simulink model "FINAL_DC_MULTIGUN_CHARGER_NEW"  (R2021b)
settings: Solver=FixedStepDiscrete  StartTime=0.0  StopTime=3600  FixedStep=0.1  RelTol=1e-3
model workspace (MAT data in the model file):
  P.stn.Ptotal_kW = 180
  P.stn.Nmod = 6
  P.stn.Pmod_kW = 30
  P.stn.Nev = 3
  P.stn.PgunMax_kW = 120
  P.stn.NmodGunMax = 4
  P.stn.Vbus_nom = 800
  P.ts.fast = 0.1
  P.ts.sup = 1
  P.tstop = 3600
  P.socStop = 0.97
  P.socMin = 0.1
  P.ev.Cap_kWh = [60 80 50]
  P.ev.Vnom = [500 560 480]
  P.ev.Vmax = [650 700 640]
  P.ev.Imax_A = [200 150 180]
  P.ev.Pmax_kW = [80 120 60]
  P.ev.Rint = [0.06 0.08 0.07]
  P.ev.SOC0 = [0.15 0.3 0.55]
  P.ev.Temp0 = [30 38 35]
  P.bms1 = '[60;500;650;200;80;0.06;30]'
  P.bms2 = '[80;560;700;150;120;0.08;38]'
  P.bms3 = '[50;480;640;180;60;0.07;35]'
  P.soc0 = [0.15; 0.3; 0.55]
  P.w.SOC = 0.35
  P.w.Demand = 0.25
  P.w.Urg = 0.25
  P.w.Fair = 0.15
  P.th.Cth = 60000
  P.th.Rth = 0.01
  P.th.Tamb = 25
  P.th.WARM = 40
  P.th.HOT = 50
  P.th.PROT = 55
  P.sw.tRampDown = 1
  P.sw.tOpenDelay = 0.2
  P.sw.tDeadTime = 0.5
  P.sw.tConnect = 0.2
  P.sw.tRampUp = 1
  P.mode = 5
  P.scenario = 2
  P.faultSchedule = 'zeros(0,4)'
settings Model: Creator=ratan  LastModifiedBy=ratan

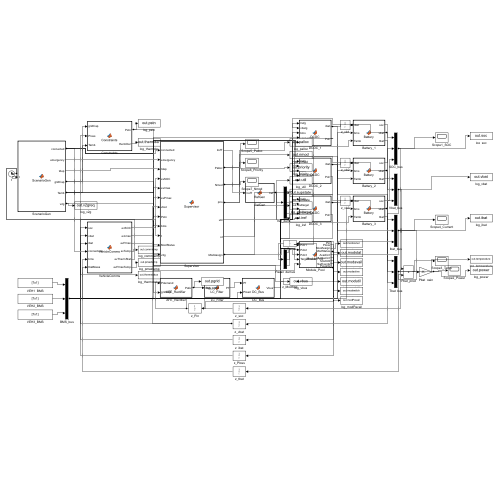
[thumbnail: Simulink's stored preview of the top-level diagram]
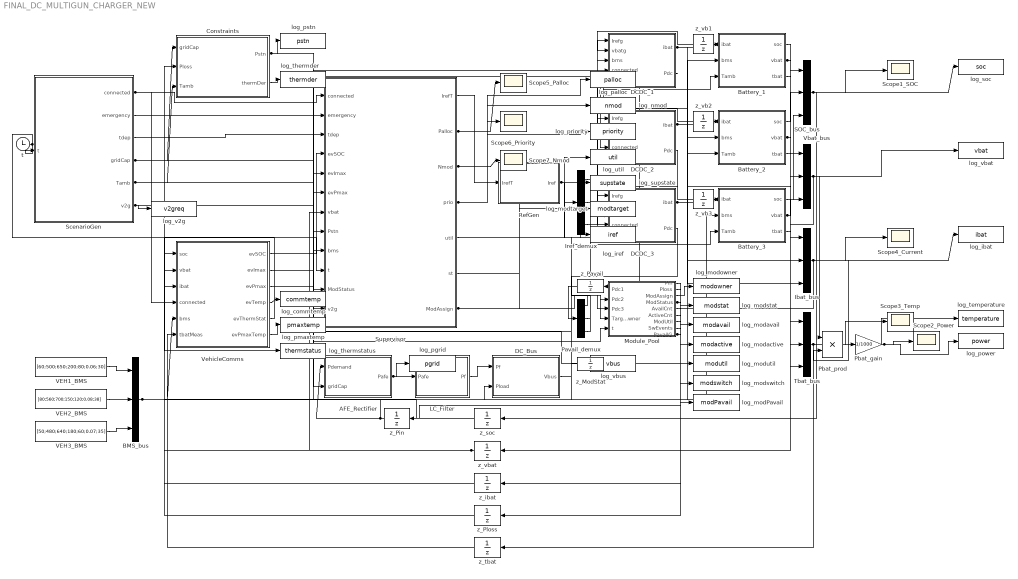
== system FINAL_DC_MULTIGUN_CHARGER_NEW ==
  AFE_Rectifier : MATLAB Function  TreatAsAtomicUnit=on
  BMS_bus : Mux  Inputs=3
  Battery_1 : MATLAB Function  TreatAsAtomicUnit=on
  Battery_2 : MATLAB Function  TreatAsAtomicUnit=on
  Battery_3 : MATLAB Function  TreatAsAtomicUnit=on
  Constraints : MATLAB Function  TreatAsAtomicUnit=on
  DCDC_1 : MATLAB Function  TreatAsAtomicUnit=on
  DCDC_2 : MATLAB Function  TreatAsAtomicUnit=on
  DCDC_3 : MATLAB Function  TreatAsAtomicUnit=on
  DC_Bus : MATLAB Function  TreatAsAtomicUnit=on
  Ibat_bus : Mux  Inputs=3
  Iref_demux : Demux  Outputs=3
  LC_Filter : MATLAB Function  TreatAsAtomicUnit=on
  Module_Pool : MATLAB Function  TreatAsAtomicUnit=on
  Pavail_demux : Demux  Outputs=3
  Pbat_gain : Gain  Gain=1/1000
  Pbat_prod : Product
  RefGen : MATLAB Function  TreatAsAtomicUnit=on
  SOC_bus : Mux  Inputs=3
  ScenarioGen : MATLAB Function  TreatAsAtomicUnit=on
  Scope1_SOC : Scope
  Scope2_Power : Scope
  Scope3_Temp : Scope
  Scope4_Current : Scope
  Scope5_Palloc : Scope
  Scope6_Priority : Scope
  Scope7_Nmod : Scope
  Supervisor : MATLAB Function  TreatAsAtomicUnit=on
  Tbat_bus : Mux  Inputs=3
  VEH1_BMS : Constant  Value=[60;500;650;200;80;0.06;30]
  VEH2_BMS : Constant  Value=[80;560;700;150;120;0.08;38]
  VEH3_BMS : Constant  Value=[50;480;640;180;60;0.07;35]
  Vbat_bus : Mux  Inputs=3
  VehicleComms : MATLAB Function  TreatAsAtomicUnit=on
  log_commtemp : ToWorkspace  VariableName=commtemp  SaveFormat=Timeseries  SampleTime=-1
  log_ibat : ToWorkspace  VariableName=ibat  SaveFormat=Timeseries  SampleTime=-1
  log_iref : ToWorkspace  VariableName=iref  SaveFormat=Timeseries  SampleTime=-1
  log_modPavail : ToWorkspace  VariableName=modPavail  SaveFormat=Timeseries  SampleTime=-1
  log_modactive : ToWorkspace  VariableName=modactive  SaveFormat=Timeseries  SampleTime=-1
  log_modavail : ToWorkspace  VariableName=modavail  SaveFormat=Timeseries  SampleTime=-1
  log_modowner : ToWorkspace  VariableName=modowner  SaveFormat=Timeseries  SampleTime=-1
  log_modstat : ToWorkspace  VariableName=modstat  SaveFormat=Timeseries  SampleTime=-1
  log_modswitch : ToWorkspace  VariableName=modswitch  SaveFormat=Timeseries  SampleTime=-1
  log_modtarget : ToWorkspace  VariableName=modtarget  SaveFormat=Timeseries  SampleTime=-1
  log_modutil : ToWorkspace  VariableName=modutil  SaveFormat=Timeseries  SampleTime=-1
  log_nmod : ToWorkspace  VariableName=nmod  SaveFormat=Timeseries  SampleTime=-1
  log_palloc : ToWorkspace  VariableName=palloc  SaveFormat=Timeseries  SampleTime=-1
  log_pgrid : ToWorkspace  VariableName=pgrid  SaveFormat=Timeseries  SampleTime=-1
  log_pmaxtemp : ToWorkspace  VariableName=pmaxtemp  SaveFormat=Timeseries  SampleTime=-1
  log_power : ToWorkspace  VariableName=power  SaveFormat=Timeseries  SampleTime=-1
  log_priority : ToWorkspace  VariableName=priority  SaveFormat=Timeseries  SampleTime=-1
  log_pstn : ToWorkspace  VariableName=pstn  SaveFormat=Timeseries  SampleTime=-1
  log_soc : ToWorkspace  VariableName=soc  SaveFormat=Timeseries  SampleTime=-1
  log_supstate : ToWorkspace  VariableName=supstate  SaveFormat=Timeseries  SampleTime=-1
  log_temperature : ToWorkspace  VariableName=temperature  SaveFormat=Timeseries  SampleTime=-1
  log_thermder : ToWorkspace  VariableName=thermder  SaveFormat=Timeseries  SampleTime=-1
  log_thermstatus : ToWorkspace  VariableName=thermstatus  SaveFormat=Timeseries  SampleTime=-1
  log_util : ToWorkspace  VariableName=util  SaveFormat=Timeseries  SampleTime=-1
  log_v2g : ToWorkspace  VariableName=v2greq  SaveFormat=Timeseries  SampleTime=-1
  log_vbat : ToWorkspace  VariableName=vbat  SaveFormat=Timeseries  SampleTime=-1
  log_vbus : ToWorkspace  VariableName=vbus  SaveFormat=Timeseries  SampleTime=-1
  t : Clock
  z_ModStat : UnitDelay  InitialCondition=[0;0;0;0;0;0]  SampleTime=0.1  HasFrameUpgradeWarning=on
  z_Pavail : UnitDelay  InitialCondition=[0;0;0]  SampleTime=0.1  HasFrameUpgradeWarning=on
  z_Pin : UnitDelay  SampleTime=0.1  HasFrameUpgradeWarning=on
  z_Ploss : UnitDelay  SampleTime=0.1  HasFrameUpgradeWarning=on
  z_ibat : UnitDelay  InitialCondition=[0;0;0]  SampleTime=0.1  HasFrameUpgradeWarning=on
  z_soc : UnitDelay  InitialCondition=[0.15;0.3;0.55]  SampleTime=0.1  HasFrameUpgradeWarning=on
  z_tbat : UnitDelay  InitialCondition=[30;38;35]  SampleTime=0.1  HasFrameUpgradeWarning=on
  z_vb1 : UnitDelay  InitialCondition=500  SampleTime=0.1  HasFrameUpgradeWarning=on
  z_vb2 : UnitDelay  InitialCondition=560  SampleTime=0.1  HasFrameUpgradeWarning=on
  z_vb3 : UnitDelay  InitialCondition=480  SampleTime=0.1  HasFrameUpgradeWarning=on
  z_vbat : UnitDelay  InitialCondition=[500;560;480]  SampleTime=0.1  HasFrameUpgradeWarning=on
  wires:
  VEH1_BMS/1 -> BMS_bus/1
  VEH2_BMS/1 -> BMS_bus/2
  VEH3_BMS/1 -> BMS_bus/3
  t/1 -> ScenarioGen/1(t), Supervisor/10(t), Module_Pool/5(t)
  ScenarioGen/1(connected) -> Supervisor/1(connected), VehicleComms/4(connected), DCDC_1/4(connected), DCDC_2/4(connected), DCDC_3/4(connected)
  ScenarioGen/2(emergency) -> Supervisor/2(emergency)
  ScenarioGen/3(tdep) -> Supervisor/3(tdep)
  ScenarioGen/6(v2g) -> Supervisor/12(v2g), log_v2g/1
  ScenarioGen/4(gridCap) -> Constraints/1(gridCap), AFE_Rectifier/2(gridCap)
  ScenarioGen/5(Tamb) -> Constraints/3(Tamb), Battery_1/3(Tamb), Battery_2/3(Tamb), Battery_3/3(Tamb)
  z_soc/1 -> VehicleComms/1(soc)
  z_vbat/1 -> VehicleComms/2(vbat), Supervisor/7(vbat)
  z_ibat/1 -> VehicleComms/3(ibat)
  BMS_bus/1 -> VehicleComms/5(bms), Supervisor/9(bms), DCDC_1/3(bms), Battery_1/2(bms), DCDC_2/3(bms), Battery_2/2(bms), DCDC_3/3(bms), Battery_3/2(bms)
  z_tbat/1 -> VehicleComms/6(tbatMeas)
  z_Ploss/1 -> Constraints/2(Ploss)
  VehicleComms/1(evSOC) -> Supervisor/4(evSOC)
  VehicleComms/2(evImax) -> Supervisor/5(evImax)
  VehicleComms/3(evPmax) -> Supervisor/6(evPmax)
  Constraints/1(Pstn) -> Supervisor/8(Pstn), log_pstn/1
  z_ModStat/1 -> Supervisor/11(ModStatus)
  Supervisor/1(IrefT) -> RefGen/1(IrefT)
  RefGen/1(Iref) -> Iref_demux/1, log_iref/1
  Iref_demux/1 -> DCDC_1/1(Irefg)
  Iref_demux/2 -> DCDC_2/1(Irefg)
  Iref_demux/3 -> DCDC_3/1(Irefg)
  Supervisor/7(ModAssign) -> Module_Pool/4(TargetOwner), log_modtarget/1
  Battery_1/2(vbat) -> z_vb1/1, Vbat_bus/1
  z_vb1/1 -> DCDC_1/2(vbatg)
  Battery_2/2(vbat) -> z_vb2/1, Vbat_bus/2
  z_vb2/1 -> DCDC_2/2(vbatg)
  Battery_3/2(vbat) -> z_vb3/1, Vbat_bus/3
  z_vb3/1 -> DCDC_3/2(vbatg)
  Pavail_demux/1 -> DCDC_1/5(Pavail)
  Pavail_demux/2 -> DCDC_2/5(Pavail)
  Pavail_demux/3 -> DCDC_3/5(Pavail)
  DCDC_1/1(ibat) -> Battery_1/1(ibat), Ibat_bus/1
  DCDC_2/1(ibat) -> Battery_2/1(ibat), Ibat_bus/2
  DCDC_3/1(ibat) -> Battery_3/1(ibat), Ibat_bus/3
  Battery_1/1(soc) -> SOC_bus/1
  Battery_2/1(soc) -> SOC_bus/2
  Battery_3/1(soc) -> SOC_bus/3
  SOC_bus/1 -> z_soc/1, Scope1_SOC/1, log_soc/1
  Vbat_bus/1 -> z_vbat/1, Pbat_prod/1, log_vbat/1
  Ibat_bus/1 -> z_ibat/1, Pbat_prod/2, Scope4_Current/1, log_ibat/1
  Battery_1/3(tbat) -> Tbat_bus/1
  Battery_2/3(tbat) -> Tbat_bus/2
  Battery_3/3(tbat) -> Tbat_bus/3
  Tbat_bus/1 -> z_tbat/1, Scope3_Temp/1, log_temperature/1
  Pbat_prod/1 -> Pbat_gain/1
  DCDC_1/2(Pdc) -> Module_Pool/1(Pdc1)
  DCDC_2/2(Pdc) -> Module_Pool/2(Pdc2)
  DCDC_3/2(Pdc) -> Module_Pool/3(Pdc3)
  Module_Pool/1(Pin) -> z_Pin/1
  Module_Pool/2(Ploss) -> z_Ploss/1
  Module_Pool/4(ModStatus) -> z_ModStat/1, log_modstat/1
  Module_Pool/9(PavailG) -> z_Pavail/1, log_modPavail/1
  z_Pavail/1 -> Pavail_demux/1
  z_Pin/1 -> AFE_Rectifier/1(Pdemand), DC_Bus/2(Pload)
  AFE_Rectifier/1(Pafe) -> LC_Filter/1(Pafe), log_pgrid/1
  LC_Filter/1(Pf) -> DC_Bus/1(Pf)
  Pbat_gain/1 -> Scope2_Power/1, log_power/1
  Supervisor/2(Palloc) -> Scope5_Palloc/1, log_palloc/1
  Supervisor/4(prio) -> Scope6_Priority/1, log_priority/1
  Supervisor/3(Nmod) -> Scope7_Nmod/1, log_nmod/1
  Supervisor/5(util) -> log_util/1
  Supervisor/6(st) -> log_supstate/1
  VehicleComms/6(evPmaxTemp) -> log_pmaxtemp/1
  VehicleComms/5(evThermStat) -> log_thermstatus/1
  VehicleComms/4(evTemp) -> log_commtemp/1
  Constraints/2(thermDer) -> log_thermder/1
  DC_Bus/1(Vbus) -> log_vbus/1
  Module_Pool/3(ModAssign) -> log_modowner/1
  Module_Pool/5(AvailCnt) -> log_modavail/1
  Module_Pool/6(ActiveCnt) -> log_modactive/1
  Module_Pool/7(ModUtil) -> log_modutil/1
  Module_Pool/8(SwEvents) -> log_modswitch/1

== matlab function FINAL_DC_MULTIGUN_CHARGER_NEW/DCDC_2 ==
  data: Irefg input; ibat output; vbatg input; bms input; connected input; Pavail input; Pdc output
function [ibat,Pdc] = DCDC(Irefg,vbatg,bms,connected,Pavail)
%#codegen
G_INJECT=2; g=G_INJECT; o=(g-1)*7;
Vmax=bms(o+3); Rint=bms(o+6); Imax=bms(o+4);
Ts=0.1; tauI=0.08; persistent I; if isempty(I), I=0; end
Icap=Pavail*1000/max(vbatg,100);
if Irefg >= 0
  Icv=max(I+(Vmax-vbatg)/max(Rint,1e-3),0);
  Icmd=min([Irefg,Icv,Icap]);
else
  Icmd=max([Irefg,-Icap,-Imax]);   % V2G discharge, magnitude-limited
end
Icmd=Icmd*(connected(g)>0.5);
I=I+(Ts/tauI)*(Icmd-I);
ibat=I; Pdc=vbatg*I/1000;
end

== matlab function FINAL_DC_MULTIGUN_CHARGER_NEW/DCDC_3 ==
  data: Irefg input; ibat output; vbatg input; bms input; connected input; Pavail input; Pdc output
function [ibat,Pdc] = DCDC(Irefg,vbatg,bms,connected,Pavail)
%#codegen
G_INJECT=3; g=G_INJECT; o=(g-1)*7;
Vmax=bms(o+3); Rint=bms(o+6); Imax=bms(o+4);
Ts=0.1; tauI=0.08; persistent I; if isempty(I), I=0; end
Icap=Pavail*1000/max(vbatg,100);
if Irefg >= 0
  Icv=max(I+(Vmax-vbatg)/max(Rint,1e-3),0);
  Icmd=min([Irefg,Icv,Icap]);
else
  Icmd=max([Irefg,-Icap,-Imax]);   % V2G discharge, magnitude-limited
end
Icmd=Icmd*(connected(g)>0.5);
I=I+(Ts/tauI)*(Icmd-I);
ibat=I; Pdc=vbatg*I/1000;
end

== matlab function FINAL_DC_MULTIGUN_CHARGER_NEW/Battery_1 ==
  data: ibat input; soc output; bms input; Tamb input; vbat output; tbat output
function [soc,vbat,tbat] = Battery(ibat,bms,Tamb)
%#codegen
G_INJECT=1; g=G_INJECT; o=(g-1)*7;
SOC0_INJECT=0.15; TBAT0_INJECT=30; CTH_INJECT=60000; RTH_INJECT=0.01;
Cap_kWh=bms(o+1); Vnom=bms(o+2); Vmax=bms(o+3); Rint=bms(o+6);
% initial SOC and initial pack temperature are scenario INITIAL CONDITIONS
% injected at build time (ov.soc0 / ov.temp0) - deliberately NOT taken from
% the runtime BMS panel, so editing VEH*_BMS cannot move the start state.
Ts=0.1; persistent SOC Tb; if isempty(SOC), SOC=SOC0_INJECT; Tb=TBAT0_INJECT; end
Ah=Cap_kWh*1000/max(Vnom,100);
SOC=min(max(SOC+ibat*Ts/3600/Ah,0),1);   % charge + discharge (V2G)
ocv=Vnom*(0.86+0.10*SOC+0.10*max(SOC-0.8,0)/0.2);
V=ocv+ibat*Rint; if V>Vmax, V=Vmax; end; if V<0.5*Vnom, V=0.5*Vnom; end
Ploss=ibat*ibat*Rint;
Tb=Tb+Ts*(Ploss-(Tb-Tamb)/max(RTH_INJECT,1e-6))/max(CTH_INJECT,1e-6);
if Tb<-30, Tb=-30; end; if Tb>90, Tb=90; end
soc=SOC; vbat=V; tbat=Tb;
end

== matlab function FINAL_DC_MULTIGUN_CHARGER_NEW/Battery_2 ==
  data: ibat input; soc output; bms input; Tamb input; vbat output; tbat output
function [soc,vbat,tbat] = Battery(ibat,bms,Tamb)
%#codegen
G_INJECT=2; g=G_INJECT; o=(g-1)*7;
SOC0_INJECT=0.3; TBAT0_INJECT=38; CTH_INJECT=60000; RTH_INJECT=0.01;
Cap_kWh=bms(o+1); Vnom=bms(o+2); Vmax=bms(o+3); Rint=bms(o+6);
% initial SOC and initial pack temperature are scenario INITIAL CONDITIONS
% injected at build time (ov.soc0 / ov.temp0) - deliberately NOT taken from
% the runtime BMS panel, so editing VEH*_BMS cannot move the start state.
Ts=0.1; persistent SOC Tb; if isempty(SOC), SOC=SOC0_INJECT; Tb=TBAT0_INJECT; end
Ah=Cap_kWh*1000/max(Vnom,100);
SOC=min(max(SOC+ibat*Ts/3600/Ah,0),1);   % charge + discharge (V2G)
ocv=Vnom*(0.86+0.10*SOC+0.10*max(SOC-0.8,0)/0.2);
V=ocv+ibat*Rint; if V>Vmax, V=Vmax; end; if V<0.5*Vnom, V=0.5*Vnom; end
Ploss=ibat*ibat*Rint;
Tb=Tb+Ts*(Ploss-(Tb-Tamb)/max(RTH_INJECT,1e-6))/max(CTH_INJECT,1e-6);
if Tb<-30, Tb=-30; end; if Tb>90, Tb=90; end
soc=SOC; vbat=V; tbat=Tb;
end

== matlab function FINAL_DC_MULTIGUN_CHARGER_NEW/Battery_3 ==
  data: ibat input; soc output; bms input; Tamb input; vbat output; tbat output
function [soc,vbat,tbat] = Battery(ibat,bms,Tamb)
%#codegen
G_INJECT=3; g=G_INJECT; o=(g-1)*7;
SOC0_INJECT=0.55; TBAT0_INJECT=35; CTH_INJECT=60000; RTH_INJECT=0.01;
Cap_kWh=bms(o+1); Vnom=bms(o+2); Vmax=bms(o+3); Rint=bms(o+6);
% initial SOC and initial pack temperature are scenario INITIAL CONDITIONS
% injected at build time (ov.soc0 / ov.temp0) - deliberately NOT taken from
% the runtime BMS panel, so editing VEH*_BMS cannot move the start state.
Ts=0.1; persistent SOC Tb; if isempty(SOC), SOC=SOC0_INJECT; Tb=TBAT0_INJECT; end
Ah=Cap_kWh*1000/max(Vnom,100);
SOC=min(max(SOC+ibat*Ts/3600/Ah,0),1);   % charge + discharge (V2G)
ocv=Vnom*(0.86+0.10*SOC+0.10*max(SOC-0.8,0)/0.2);
V=ocv+ibat*Rint; if V>Vmax, V=Vmax; end; if V<0.5*Vnom, V=0.5*Vnom; end
Ploss=ibat*ibat*Rint;
Tb=Tb+Ts*(Ploss-(Tb-Tamb)/max(RTH_INJECT,1e-6))/max(CTH_INJECT,1e-6);
if Tb<-30, Tb=-30; end; if Tb>90, Tb=90; end
soc=SOC; vbat=V; tbat=Tb;
end

== matlab function FINAL_DC_MULTIGUN_CHARGER_NEW/Module_Pool ==
  data: Pdc1 input; Pin output; Pdc2 input; Pdc3 input; TargetOwner input; t input; Ploss output; ModAssign output; ModStatus output; AvailCnt output; ActiveCnt output; ModUtil output; SwEvents output; PavailG output
function [Pin,Ploss,ModAssign,ModStatus,AvailCnt,ActiveCnt,ModUtil,SwEvents,PavailG] = ModulePool(Pdc1,Pdc2,Pdc3,TargetOwner,t)
%#codegen
Pmod=30; eta=0.955; SWLOSS_KW=0.3;
TRD_M=1; TOPEN_M=0.2; TDEAD_M=0.5; TCONN_M=0.2; TRUP_M=1;
FAULT_SCHEDULE=zeros(0,4); Ts=0.1;
persistent owner phase timer contrib pend swCnt initMP;
if isempty(initMP), owner=zeros(6,1); phase=zeros(6,1); timer=zeros(6,1); contrib=zeros(6,1); pend=zeros(6,1); swCnt=0; initMP=1; end
health=zeros(6,1);
for r=1:size(FAULT_SCHEDULE,1), mid=FAULT_SCHEDULE(r,1); if t>=FAULT_SCHEDULE(r,2) && t<=FAULT_SCHEDULE(r,3), health(mid)=FAULT_SCHEDULE(r,4); end, end
for id=1:6
  tgt=TargetOwner(id);
  if health(id)~=0
    owner(id)=0; pend(id)=0; contrib(id)=0;
    if phase(id)~=0, timer(id)=timer(id)+Ts; if timer(id)>=TDEAD_M, phase(id)=0; timer(id)=0; end, end
  else
    switch phase(id)
      case 0, if tgt>0, pend(id)=tgt; phase(id)=5; timer(id)=0; end
      case 1, if tgt~=owner(id), pend(id)=tgt; phase(id)=2; timer(id)=0; end
      case 2, timer(id)=timer(id)+Ts; contrib(id)=max(1-timer(id)/max(TRD_M,1e-3),0); if timer(id)>=TRD_M, phase(id)=3; timer(id)=0; contrib(id)=0; end
      case 3, timer(id)=timer(id)+Ts; if timer(id)>=TOPEN_M, owner(id)=0; phase(id)=4; timer(id)=0; end
      case 4, timer(id)=timer(id)+Ts; if timer(id)>=TDEAD_M, if pend(id)>0, phase(id)=5; timer(id)=0; else phase(id)=0; timer(id)=0; end, end
      case 5, timer(id)=timer(id)+Ts; if timer(id)>=TCONN_M, owner(id)=pend(id); pend(id)=0; phase(id)=6; timer(id)=0; end
      case 6, timer(id)=timer(id)+Ts; contrib(id)=min(timer(id)/max(TRUP_M,1e-3),1); if timer(id)>=TRUP_M, phase(id)=1; timer(id)=0; contrib(id)=1; swCnt=swCnt+1; end
    end
  end
end
ModAssign=owner; ModUtil=contrib; ModStatus=zeros(6,1);
for id=1:6, if health(id)~=0, ModStatus(id)=health(id)+1; elseif phase(id)==0, ModStatus(id)=0; else ModStatus(id)=1; end, end
AvailCnt=sum(ModStatus==0); ActiveCnt=sum(phase>0 & health==0); SwEvents=swCnt;
PavailG=zeros(3,1); for id=1:6, gg=owner(id); if gg>0, PavailG(gg)=PavailG(gg)+contrib(id)*Pmod; end, end
nTrans=sum(phase>=2 & phase<=5 & health==0);
Pdc=Pdc1+Pdc2+Pdc3;
if Pdc>=0, Pin=Pdc/eta+SWLOSS_KW*nTrans; else Pin=Pdc*eta+SWLOSS_KW*nTrans; end
Ploss=abs(Pin-Pdc);
end

== matlab function FINAL_DC_MULTIGUN_CHARGER_NEW/AFE_Rectifier ==
  data: Pdemand input; Pafe output; gridCap input
function Pafe = AFE_Rectifier(Pdemand,gridCap)
%#codegen
Ts=0.1; SLEW=60; persistent P; if isempty(P), P=0; end
tgt=min(Pdemand,gridCap);   % gridCap limits import; export (negative) passes
P=P+max(min(tgt-P,SLEW*Ts),-SLEW*Ts);
Pafe=P;   % may be negative (V2G export to grid)
end

== matlab function FINAL_DC_MULTIGUN_CHARGER_NEW/LC_Filter ==
  data: Pafe input; Pf output
function Pf = LC_Filter(Pafe)
%#codegen
Ts=0.1; tau=0.3; persistent P; if isempty(P), P=0; end
P=P+(Ts/tau)*(Pafe-P); Pf=P;
end

== matlab function FINAL_DC_MULTIGUN_CHARGER_NEW/DC_Bus ==
  data: Pf input; Vbus output; Pload input
function Vbus = DC_Bus(Pf,Pload)
%#codegen
Ts=0.1; Cbus=0.12; Vnom=800; persistent Vb; if isempty(Vb), Vb=Vnom; end
Vb=Vb+Ts*(Pf-Pload)*1000/(Cbus*max(Vb,400)); Vb=min(max(Vb,400),900); Vbus=Vb;
end

== matlab function FINAL_DC_MULTIGUN_CHARGER_NEW/VehicleComms ==
  data: soc input; evSOC output; vbat input; ibat input; connected input; bms input; tbatMeas input; evImax output; evPmax output; evTemp output; evThermStat output; evPmaxTemp output
function [evSOC,evImax,evPmax,evTemp,evThermStat,evPmaxTemp] = VehicleComms(soc,vbat,ibat,connected,bms,tbatMeas) %#ok<INUSD>
%#codegen
SOC0_VEC = [0.15;0.3;0.55];
ImaxRaw = [bms(4); bms(11); bms(18)];
PmaxRaw = [bms(5); bms(12); bms(19)];
VmaxV   = [bms(3); bms(10); bms(17)];
TbmsV   = [bms(7); bms(14); bms(21)];
TempV = tbatMeas;
for g=1:3, if ~isfinite(TempV(g))||TempV(g)<=-50, TempV(g)=TbmsV(g); end, end
thermFac = ones(3,1); ThermStat = zeros(3,1);
for g=1:3
  T = TempV(g);
  if T >= 55
    thermFac(g)=0;    ThermStat(g)=3;   % PROTECTION
  elseif T >= 50
    thermFac(g)=0.40; ThermStat(g)=2;   % HOT
  elseif T >= 40
    thermFac(g)=0.70; ThermStat(g)=1;   % WARM
  else
    thermFac(g)=1.00; ThermStat(g)=0;   % NORMAL
  end
end
ImaxV = ImaxRaw .* thermFac;
PmaxV = PmaxRaw .* thermFac;
DLY = 2; persistent bufS bufI bufP w;
if isempty(bufS), bufS=repmat(SOC0_VEC,1,DLY+1); bufI=repmat(ImaxV,1,DLY+1); bufP=repmat(PmaxV,1,DLY+1); w=1; end
Iacc=zeros(3,1); Pacc=zeros(3,1);
for g=1:3
  if connected(g)>0.5
    head=max(VmaxV(g)-vbat(g),0);
    Iacc(g)=ImaxV(g)*min(head/25,1);
    Pacc(g)=min(PmaxV(g),Iacc(g)*vbat(g)/1000);
  end
end
bufS(:,w)=soc; bufI(:,w)=Iacc; bufP(:,w)=Pacc;
r=w+1; if r>DLY+1, r=1; end
evSOC=bufS(:,r); evImax=bufI(:,r); evPmax=bufP(:,r); w=r;
evTemp=TempV; evThermStat=ThermStat; evPmaxTemp=PmaxV;
end

== matlab function FINAL_DC_MULTIGUN_CHARGER_NEW/ScenarioGen ==
  data: t input; connected output; emergency output; tdep output; gridCap output; Tamb output; v2g output
function [connected,emergency,tdep,gridCap,Tamb,v2g] = ScenarioGen(t)
%#codegen
CONN0 = [1;1;1];
TDEP = [3400;3000;3400];
V2GREQ = [0;0;0];
TAMB = 25;
GC0 = 180; GCLO = 180; GT0 = 1000000000; GT1 = 1000000000;
DISCEV = 0; DISCT = 1000000000;
LATEEV = 0; LATET = 0;
connected = CONN0;
if LATEEV>=1 && LATEEV<=3 && t < LATET, connected(LATEEV) = 0; end
if DISCEV>=1 && DISCEV<=3 && t >= DISCT, connected(DISCEV) = 0; end
gridCap = GC0; if t >= GT0 && t < GT1, gridCap = GCLO; end
Tamb = TAMB;
tdep = TDEP;
v2g = V2GREQ .* (connected > 0.5);
emergency = zeros(3,1);
end

== matlab function FINAL_DC_MULTIGUN_CHARGER_NEW/Constraints ==
  data: gridCap input; Pstn output; Ploss input; Tamb input; thermDer output
function [Pstn,thermDer] = Constraints(gridCap,Ploss,Tamb)
%#codegen
Ptotal=180; Ts=1.0; RAMP=10;
persistent PgridF Tcab derOn;
if isempty(PgridF), PgridF=Ptotal; Tcab=Tamb; derOn=0; end
PgridF=PgridF+max(min(gridCap-PgridF,RAMP*Ts),-RAMP*Ts);
Rth=0.045; Cth=400;
Tcab=Tcab+(Ts/Cth)*(max(Ploss,0)-(Tcab-Tamb)/Rth)*Rth;
if derOn==0 && Tcab>75, derOn=1; end
if derOn==1 && Tcab<65, derOn=0; end
if derOn==1, thermDer=max(0.4,1-0.03*(Tcab-75)); else thermDer=1.0; end
Pstn=min(PgridF,Ptotal)*thermDer;
end

== matlab function FINAL_DC_MULTIGUN_CHARGER_NEW/Supervisor ==
  data: connected input; IrefT output; emergency input; tdep input; evSOC input; evImax input; evPmax input; vbat input; Pstn input; bms input; t input; ModStatus input; v2g input; Palloc output; Nmod output; prio output; util output; st output; ModAssign output
function [IrefT,Palloc,Nmod,prio,util,st,ModAssign] = Supervisor(connected,emergency,tdep,evSOC,evImax,evPmax,vbat,Pstn,bms,t,ModStatus,v2g)
%#codegen
MODE_INJECT = 5; mode = MODE_INJECT;
Pmod=30; NmodTot=6; NmodGunMax=4; PgunMax=120; socMin=0.10;
Cap_kWh=[bms(1);bms(8);bms(15)]; PmaxV=[bms(5);bms(12);bms(19)]; ImaxV=[bms(4);bms(11);bms(18)];
soc_stop=0.97; Ts=1.0; tauF=30; DB=0.25; TDWELL=60; TSUST=20; TRD=2; TSW=3; MARGIN=5;
wS=0.35; wD=0.25; wU=0.25; wF=0.15;
persistent prioF modMap pendMap ordP tLast reSt reT taperC Edel swCnt lastC lastP modOwner init;
if isempty(init)
  prioF=zeros(3,1); modMap=zeros(3,1); pendMap=zeros(3,1); ordP=[1;2;3]; tLast=-1e9;
  reSt=0; reT=0; taperC=zeros(3,1); Edel=zeros(3,1); swCnt=0; lastC=zeros(3,1); lastP=180; modOwner=zeros(6,1); init=1;
end
IrefT=zeros(3,1); Palloc=zeros(3,1); prio=zeros(3,1);
% ---- classify: export (V2G) vs charge (G2V) -----------------------
isExp=zeros(3,1); active=zeros(3,1); Pacc=zeros(3,1);
for g=1:3
  if connected(g)>0.5 && v2g(g)>0.5 && evSOC(g)>socMin
    isExp(g)=1; active(g)=1; Pacc(g)=min([v2g(g),PgunMax,PmaxV(g)]);
  elseif connected(g)>0.5 && evSOC(g)<soc_stop && evPmax(g)>1
    active(g)=1; Pacc(g)=min(evPmax(g),PgunMax);
  end
end
% ---- equal-finish-time SOFT sizing (G2V only) ---------------------
Pdes=Pacc; Eneed=zeros(3,1);
for g=1:3, if active(g)>0.5 && isExp(g)<0.5, Eneed(g)=Cap_kWh(g)*max(soc_stop-evSOC(g),0); end, end
if sum(Eneed)>1e-3
  Tstar=sum(Eneed)/max(Pstn,1e-3);
  for g=1:3, if active(g)>0.5 && isExp(g)<0.5 && Pacc(g)>1, Tstar=max(Tstar,Eneed(g)/Pacc(g)); end, end
  for g=1:3, if active(g)>0.5 && isExp(g)<0.5, Pdes(g)=min(Eneed(g)/max(Tstar,1e-4),Pacc(g)); end, end
end
% ---- priority score (fixed weights) -------------------------------
Etot=max(sum(Edel),1e-6);
for g=1:3
  if active(g)>0.5
    if isExp(g)>0.5
      prio(g)=0.5 + 10*emergency(g);   % V2G mid priority for module claim
    else
      S=1-evSOC(g); D=min(Pdes(g)/PgunMax,1); trem=max(tdep(g)-t,60)/3600;
      U=min(Cap_kWh(g)*(soc_stop-evSOC(g))/max(evPmax(g)*trem,1e-3),2); F=1-Edel(g)/Etot;
      prio(g)=wS*S+wD*D+wU*U+wF*F+10*emergency(g);
    end
  end
end
prioF=prioF+(Ts/tauF)*(prio-prioF);
for k=1:2, a=ordP(k); b=ordP(k+1); if prioF(b)>prioF(a)+DB, ordP(k)=b; ordP(k+1)=a; end, end
% ---- events -------------------------------------------------------
evPlug=any(abs(connected-lastC)>0.5); evDer=abs(Pstn-lastP)>5; evTap=0;
for g=1:3
  if modMap(g)>1 && active(g)>0.5 && Pdes(g)<(modMap(g)-1)*Pmod-MARGIN
    taperC(g)=taperC(g)+Ts; if taperC(g)>TSUST, evTap=1; end
  else, taperC(g)=0; end
end
dwellOK=(t-tLast)>TDWELL; forced=evPlug; wantRe=forced||(dwellOK&&(evDer||evTap));
% ---- target module map (event-driven) -----------------------------
if reSt==0 && wantRe
  tgt=zeros(3,1); left=NmodTot;
  for k=1:3, g=ordP(k); if active(g)>0.5 && tgt(g)==0 && left>0, tgt(g)=1; left=left-1; end, end
  for k=1:3, g=ordP(k);
    if active(g)>0.5, nWant=min(ceil(Pdes(g)/Pmod),NmodGunMax); add=min(nWant-tgt(g),left); if add>0, tgt(g)=tgt(g)+add; left=left-add; end, end
  end
  adopt=1;
  if ~forced
    oldDel=0; newDel=0;
    for g=1:3, oldDel=oldDel+min(modMap(g)*Pmod,Pdes(g)); newDel=newDel+min(tgt(g)*Pmod,Pdes(g)); end
    if (newDel-oldDel)<Pmod && evTap==0, adopt=0; end
  end
  if adopt && any(tgt~=modMap)
    pendMap=tgt;
    if all(tgt>=modMap), swCnt=swCnt+sum(abs(tgt-modMap)); modMap=tgt; tLast=t; taperC=zeros(3,1);
    else reSt=1; reT=0; end
  end
end
if reSt==1, reT=reT+Ts; if reT>=TRD, reSt=2; reT=0; end
elseif reSt==2, reT=reT+Ts; if reT>=TSW, swCnt=swCnt+sum(abs(pendMap-modMap)); modMap=pendMap; tLast=t; taperC=zeros(3,1); reSt=0; reT=0; end
end
% ---- power within module ceilings + station limit -----------------
ceilP=zeros(3,1);
for g=1:3, n=modMap(g); if reSt>0 && pendMap(g)<modMap(g), n=pendMap(g); end, ceilP(g)=min(n*Pmod,PgunMax); end
for g=1:3, Palloc(g)=min(ceilP(g),Pdes(g)); end
drawSum=0; for g=1:3, if isExp(g)<0.5, drawSum=drawSum+Palloc(g); end, end
if drawSum>Pstn && drawSum>0, sc=Pstn/drawSum; for g=1:3, if isExp(g)<0.5, Palloc(g)=Palloc(g)*sc; end, end, end
left=Pstn-drawSum;
for k=1:3, g=ordP(k); if left<=0, break; end, if isExp(g)<0.5, room=min(ceilP(g),Pacc(g))-Palloc(g); give=min(room,left); if give>0, Palloc(g)=Palloc(g)+give; left=left-give; end, end, end
% ---- current targets (sign preserved) -----------------------------
for g=1:3
  if isExp(g)>0.5
    Palloc(g)=-Palloc(g);
    IrefT(g)=-min(abs(Palloc(g))*1000/max(vbat(g),100),ImaxV(g));
  elseif Palloc(g)>0
    IrefT(g)=min(Palloc(g)*1000/max(vbat(g),100),evImax(g));
  end
end
% ---- bookkeeping --------------------------------------------------
Edel=Edel+abs(Palloc)*(Ts/3600); lastC=connected; lastP=Pstn; Nmod=modMap;
Ptot=0; for g=1:3, Ptot=Ptot+abs(Palloc(g)); end
util=[Ptot; 100*Ptot/max(Pstn,1e-6); Pstn-Ptot]; st=[reSt; swCnt; max(TDWELL-(t-tLast),0)];
% ---- module-ID assignment (fault-aware) ---------------------------
for id=1:6, if ModStatus(id)>=2 && modOwner(id)~=0, modOwner(id)=0; end, end
curCnt=zeros(3,1); for g=1:3, curCnt(g)=sum(modOwner==g); end
for g=1:3, ex=curCnt(g)-modMap(g); if ex>0, for id=6:-1:1, if ex<=0, break; end, if modOwner(id)==g, modOwner(id)=0; ex=ex-1; end, end, end, end
for g=1:3, curCnt(g)=sum(modOwner==g); end
for k=1:3, g=ordP(k); need=modMap(g)-curCnt(g); if need>0, for id=1:6, if need<=0, break; end, if modOwner(id)==0 && ModStatus(id)==0, modOwner(id)=g; need=need-1; end, end, end, end
ModAssign=modOwner;
end

== matlab function FINAL_DC_MULTIGUN_CHARGER_NEW/RefGen ==
  data: IrefT input; Iref output
function Iref = RefGen(IrefT)
%#codegen
Ts=0.1; UP=20; DOWN=100;
persistent I; if isempty(I), I=zeros(3,1); end
for g=1:3
  d=IrefT(g)-I(g);
  I(g)=I(g)+max(min(d,UP*Ts),-DOWN*Ts);
end
Iref=I;   % negative allowed for V2G (no clamp to zero)
end

== matlab function FINAL_DC_MULTIGUN_CHARGER_NEW/DCDC_1 ==
  data: Irefg input; ibat output; vbatg input; bms input; connected input; Pavail input; Pdc output
function [ibat,Pdc] = DCDC(Irefg,vbatg,bms,connected,Pavail)
%#codegen
G_INJECT=1; g=G_INJECT; o=(g-1)*7;
Vmax=bms(o+3); Rint=bms(o+6); Imax=bms(o+4);
Ts=0.1; tauI=0.08; persistent I; if isempty(I), I=0; end
Icap=Pavail*1000/max(vbatg,100);
if Irefg >= 0
  Icv=max(I+(Vmax-vbatg)/max(Rint,1e-3),0);
  Icmd=min([Irefg,Icv,Icap]);
else
  Icmd=max([Irefg,-Icap,-Imax]);   % V2G discharge, magnitude-limited
end
Icmd=Icmd*(connected(g)>0.5);
I=I+(Ts/tauI)*(Icmd-I);
ibat=I; Pdc=vbatg*I/1000;
end
